simulink model "disturbed_roll_system"  (R2019b)
settings: Solver=VariableStepAuto  StartTime=0.0  StopTime=4  RelTol=1e-3
undefined symbols (not defined in the file or in its folder): G_phi_samples
libraries: simulink x12, cstblocks x5
settings Model: Creator=amirhossein  LastModifiedBy=amirhossein

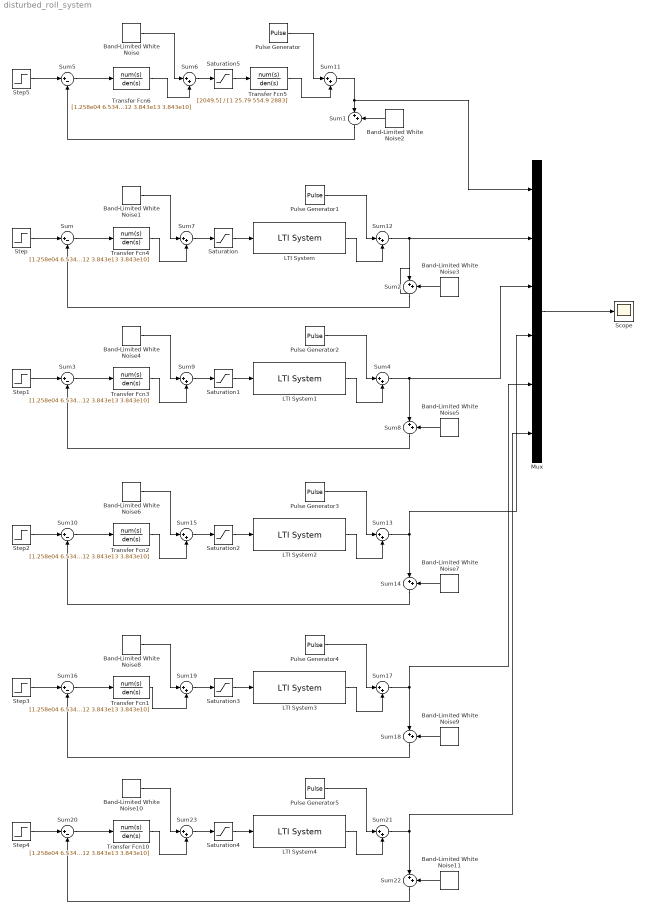
== system disturbed_roll_system ==
  Band-Limited White Noise{,1,4,6,8,10} (6 alike) : simulink/Sources/Band-Limited White Noise  Cov=[0.001]  Ts=0.01  seed=[23341]
  Band-Limited White Noise{2..3,5,7,9,11} (6 alike) : simulink/Sources/Band-Limited White Noise  Cov=[0.0001]  Ts=0.01  seed=[23341]
  LTI System : cstblocks/LTI System  sys=G_phi_samples(: , : , 1)  IC=[]
  LTI System1 : cstblocks/LTI System  sys=G_phi_samples(: , : , 2)  IC=[]
  LTI System2 : cstblocks/LTI System  sys=G_phi_samples(: , : , 3)  IC=[]
  LTI System3 : cstblocks/LTI System  sys=G_phi_samples(: , : , 4)  IC=[]
  LTI System4 : cstblocks/LTI System  sys=G_phi_samples(: , : , 5)  IC=[]
  Mux : Mux  Inputs=6
  Pulse Generator{,1..5} (6 alike) : DiscretePulseGenerator  PulseType=Time based  Amplitude=0.1  Period=1.5  PulseWidth=5
  Saturation{,1..5} (6 alike) : Saturate  UpperLimit=20  LowerLimit=-20
  Scope : Scope
  Step{,1..5} (6 alike) : Step  SampleTime=0
  Sum{,3,5,10,16,20} (6 alike) : Sum  Inputs=|+-
  Sum{1..2,4,6..9,11..15,17..19,21..23} (18 alike) : Sum  Inputs=|++
  Transfer Fcn{1..4,6,10} (6 alike) : TransferFcn  Numerator=[1.258e04 6.534e06 6.665e08 3.016e10 7.851e11 1.256e13 1.142e14 3.868e14]  Denominator=[1 2032 1.172e06 1.496e08 9.86e09 3.484e11 5.991e12 3.843e13 3.843e10]
  Transfer Fcn5 : TransferFcn  Numerator=[2049.5]  Denominator=[1 25.79 554.9 2883]
  wires:
  Sum16/1 -> Transfer Fcn1/1
  Pulse Generator1/1 -> Sum12/1
  Sum8/1 -> Sum3/2
  Sum12/1 -> Sum2/1, Mux/2
  Step4/1 -> Sum20/1
  Sum19/1 -> Saturation3/1
  Band-Limited White Noise8/1 -> Sum19/1
  Sum5/1 -> Transfer Fcn6/1
  Transfer Fcn4/1 -> Sum7/2
  LTI System2/1 -> Sum13/2
  Sum6/1 -> Saturation5/1
  Sum10/1 -> Transfer Fcn2/1
  LTI System/1 -> Sum12/2
  Saturation5/1 -> Transfer Fcn5/1
  Transfer Fcn6/1 -> Sum6/2
  Step/1 -> Sum/1
  Saturation4/1 -> LTI System4/1
  Saturation3/1 -> LTI System3/1
  Transfer Fcn1/1 -> Sum19/2
  LTI System4/1 -> Sum21/2
  Sum13/1 -> Mux/4, Sum14/1
  Band-Limited White Noise6/1 -> Sum15/1
  Sum20/1 -> Transfer Fcn10/1
  Transfer Fcn3/1 -> Sum9/2
  Transfer Fcn2/1 -> Sum15/2
  Pulse Generator5/1 -> Sum21/1
  LTI System3/1 -> Sum17/2
  Saturation2/1 -> LTI System2/1
  Saturation/1 -> LTI System/1
  Pulse Generator4/1 -> Sum17/1
  Band-Limited White Noise11/1 -> Sum22/2
  Step5/1 -> Sum5/1
  Sum15/1 -> Saturation2/1
  Sum23/1 -> Saturation4/1
  Band-Limited White Noise3/1 -> Sum2/2
  Band-Limited White Noise10/1 -> Sum23/1
  Step3/1 -> Sum16/1
  Sum4/1 -> Mux/3, Sum8/1
  Sum11/1 -> Sum1/1, Mux/1
  Transfer Fcn10/1 -> Sum23/2
  Band-Limited White Noise9/1 -> Sum18/2
  Sum/1 -> Transfer Fcn4/1
  Band-Limited White Noise/1 -> Sum6/1
  Step2/1 -> Sum10/1
  Sum17/1 -> Mux/5, Sum18/1
  Pulse Generator/1 -> Sum11/1
  Band-Limited White Noise7/1 -> Sum14/2
  Sum21/1 -> Mux/6, Sum22/1
  Transfer Fcn5/1 -> Sum11/2
  Sum14/1 -> Sum10/2
  Pulse Generator3/1 -> Sum13/1
  Pulse Generator2/1 -> Sum4/1
  Band-Limited White Noise1/1 -> Sum7/1
  Sum1/1 -> Sum5/2
  LTI System1/1 -> Sum4/2
  Band-Limited White Noise5/1 -> Sum8/2
  Saturation1/1 -> LTI System1/1
  Band-Limited White Noise4/1 -> Sum9/1
  Sum3/1 -> Transfer Fcn3/1
  Sum9/1 -> Saturation1/1
  Sum18/1 -> Sum16/2
  Sum22/1 -> Sum20/2
  Step1/1 -> Sum3/1
  Sum7/1 -> Saturation/1
  Sum2/1 -> Sum/2
  Band-Limited White Noise2/1 -> Sum1/2
  Mux/1 -> Scope/1
